simulink model "DynamicModel"  (R2022b)
settings: Solver=VariableStepAuto  StartTime=0.0  StopTime=t  FixedStep=t / k
values from neighbouring files (symbols this model uses):
  dq_0 = zeros(3, 1)    [USA_WPI.m]
  I1_n = 0.5 * (I1_n + I1_n')    [USA_WPI.m]
  I2_n = 0.5 * (I2_n + I2_n')    [USA_WPI.m]
  I3_n = 0.5 * (I3_n + I3_n')    [USA_WPI.m]
  Kp = 10 * eye(3)    [USA_WPI.m]
  L_n = [0 0.64 0.96]    [USA_WPI.m]
  Lcom_n = L_n / 2    [USA_WPI.m]
  m_n = [29.1735 40.0393 22.3124]    [USA_WPI.m]
  q_0 = randn(3, 1)    [USA_WPI.m]
settings Model: Creator=mluser  LastModifiedBy=Gary-pc
settings DataIOCC: ExternalInput=q1_s, q2_s, q3_s, dq1_s, dq2_s, dq3_s, ddq1_s, ddq2_s, ddq3_s  LoadExternalInput=on  SaveOutput=off  SignalLogging=off  DSMLogging=off  SaveTime=off  ReturnWorkspaceOutputs=off
settings ModelReferenceCC: EnableRefExpFcnMdlSchedulingChecks=on

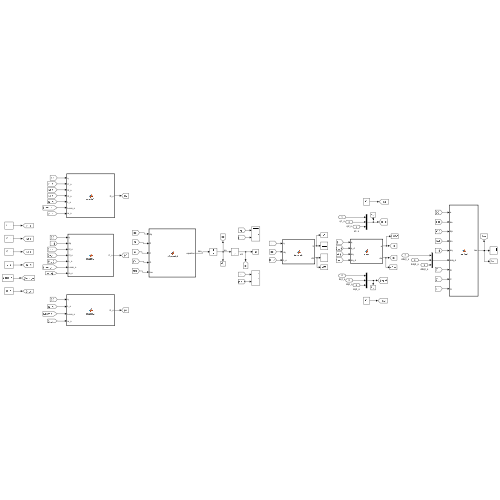
[thumbnail: Simulink's stored preview of the top-level diagram]
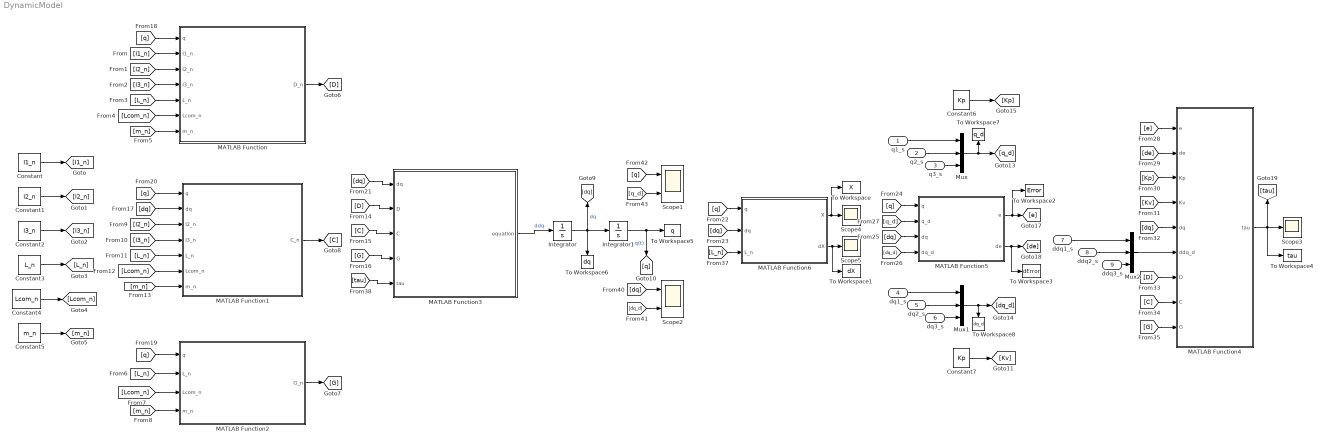
== system DynamicModel ==
  q1_s : Inport
  q2_s : Inport  Port=2
  q3_s : Inport  Port=3
  dq1_s : Inport  Port=4
  dq2_s : Inport  Port=5
  dq3_s : Inport  Port=6
  ddq1_s : Inport  Port=7
  ddq2_s : Inport  Port=8
  ddq3_s : Inport  Port=9
  Constant : Constant  Value=I1_n
  Constant1 : Constant  Value=I2_n
  Constant2 : Constant  Value=I3_n
  Constant3 : Constant  Value=L_n
  Constant4 : Constant  Value=Lcom_n
  Constant5 : Constant  Value=m_n
  Constant6 : Constant  Value=Kp
  Constant7 : Constant  Value=Kp
  Integrator : Integrator  InitialCondition=dq_0
  Integrator1 : Integrator  InitialCondition=q_0
  MATLAB Function : MATLAB Function  TreatAsAtomicUnit=on
  MATLAB Function1 : MATLAB Function  TreatAsAtomicUnit=on
  MATLAB Function2 : MATLAB Function  TreatAsAtomicUnit=on
  MATLAB Function3 : MATLAB Function  TreatAsAtomicUnit=on
  MATLAB Function4 : MATLAB Function  TreatAsAtomicUnit=on
  MATLAB Function5 : MATLAB Function  TreatAsAtomicUnit=on
  MATLAB Function6 : MATLAB Function  TreatAsAtomicUnit=on
  Mux : Mux  Inputs=3
  Mux1 : Mux  Inputs=3
  Mux2 : Mux  Inputs=3
  Scope1 : Scope  NumInputPorts=2
  Scope2 : Scope  NumInputPorts=2
  Scope3 : Scope
  Scope4 : Scope
  Scope5 : Scope
  To Workspace : ToWorkspace  VariableName=X  SaveFormat=Timeseries  SampleTime=-1
  To Workspace1 : ToWorkspace  VariableName=dX  SaveFormat=Timeseries  SampleTime=-1
  To Workspace2 : ToWorkspace  VariableName=Error  SaveFormat=Timeseries  SampleTime=-1
  To Workspace3 : ToWorkspace  VariableName=dError  SaveFormat=Timeseries  SampleTime=-1
  To Workspace4 : ToWorkspace  VariableName=tau  SaveFormat=Timeseries  SampleTime=-1
  To Workspace5 : ToWorkspace  VariableName=q  SaveFormat=Timeseries  SampleTime=-1
  To Workspace6 : ToWorkspace  VariableName=dq  SaveFormat=Timeseries  SampleTime=-1
  To Workspace7 : ToWorkspace  VariableName=q_d  SaveFormat=Timeseries  SampleTime=-1
  To Workspace8 : ToWorkspace  VariableName=dq_d  SaveFormat=Timeseries  SampleTime=-1
  wires:
  Integrator/1 -> To Workspace6/1, [dq], Integrator1/1  "dq"
  Integrator1/1 -> To Workspace5/1, [q]  "q(t)"
  Constant/1 -> [I1_n]
  Constant1/1 -> [I2_n]
  Constant2/1 -> [I3_n]
  Constant3/1 -> [L_n]
  Constant4/1 -> [Lcom_n]
  Constant5/1 -> [m_n]
  [I1_n] -> MATLAB Function/2(I1_n)
  [I2_n] -> MATLAB Function/3(I2_n)
  [I3_n] -> MATLAB Function/4(I3_n)
  [L_n] -> MATLAB Function/5(L_n)
  [Lcom_n] -> MATLAB Function/6(Lcom_n)
  [m_n] -> MATLAB Function/7(m_n)
  [I2_n] -> MATLAB Function1/3(I2_n)
  [I3_n] -> MATLAB Function1/4(I3_n)
  [L_n] -> MATLAB Function1/5(L_n)
  [Lcom_n] -> MATLAB Function1/6(Lcom_n)
  [m_n] -> MATLAB Function1/7(m_n)
  MATLAB Function3/1(equation) -> Integrator/1  "ddq"
  MATLAB Function/1(D_n) -> [D]
  MATLAB Function2/1(G_n) -> [G]
  MATLAB Function1/1(C_n) -> [C]
  [D] -> MATLAB Function3/2(D)
  [C] -> MATLAB Function3/3(C)
  [G] -> MATLAB Function3/4(G)
  [dq] -> MATLAB Function1/2(dq)
  [q] -> MATLAB Function/1(q)
  [q] -> MATLAB Function1/1(q)
  [dq] -> MATLAB Function3/1(dq)
  [q] -> MATLAB Function2/1(q)
  [L_n] -> MATLAB Function2/2(L_n)
  [Lcom_n] -> MATLAB Function2/3(Lcom_n)
  [m_n] -> MATLAB Function2/4(m_n)
  [q] -> MATLAB Function5/1(q)
  [dq] -> MATLAB Function5/3(dq)
  [dq_d] -> MATLAB Function5/4(dq_d)
  [q_d] -> MATLAB Function5/2(q_d)
  MATLAB Function5/1(e) -> To Workspace2/1, [e]
  MATLAB Function5/2(de) -> To Workspace3/1, [de]
  [e] -> MATLAB Function4/1(e)
  [de] -> MATLAB Function4/2(de)
  [Kp] -> MATLAB Function4/3(Kp)
  [Kv] -> MATLAB Function4/4(Kv)
  [dq] -> MATLAB Function4/5(dq)
  [D] -> MATLAB Function4/7(D)
  [C] -> MATLAB Function4/8(C)
  [G] -> MATLAB Function4/9(G)
  [tau] -> MATLAB Function3/5(tau)
  [dq] -> Scope2/1
  [dq_d] -> Scope2/2
  [q] -> Scope1/1
  [q_d] -> Scope1/2
  MATLAB Function4/1(tau) -> To Workspace4/1, Scope3/1, [tau]
  q1_s/1 -> Mux/1
  q2_s/1 -> Mux/2
  q3_s/1 -> Mux/3
  Mux/1 -> To Workspace7/1, [q_d]
  dq3_s/1 -> Mux1/3
  dq1_s/1 -> Mux1/1
  dq2_s/1 -> Mux1/2
  ddq2_s/1 -> Mux2/2
  ddq1_s/1 -> Mux2/1
  Mux2/1 -> MATLAB Function4/6(ddq_d)
  ddq3_s/1 -> Mux2/3
  Constant6/1 -> [Kp]
  Constant7/1 -> [Kv]
  [q] -> MATLAB Function6/1(q)
  [L_n] -> MATLAB Function6/3(L_n)
  [dq] -> MATLAB Function6/2(dq)
  MATLAB Function6/1(X) -> To Workspace/1, Scope4/1
  MATLAB Function6/2(dX) -> To Workspace1/1, Scope5/1
  Mux1/1 -> To Workspace8/1, [dq_d]

== matlab function DynamicModel/MATLAB Function1 ==
  data: C_n output; q input; dq input; I2_n input; I3_n input; L_n input; Lcom_n input; m_n input
function C_n = matrixC(q, dq, I2_n, I3_n, L_n, Lcom_n, m_n)

%% Evaluate anonymous function
C_n = functionC(I2_n(1, 1), ...
                I3_n(1, 1), ...
                I2_n(1, 2), ...
                I3_n(1, 2), ...
                I2_n(1, 3), ...
                I3_n(1, 3), ...
                I2_n(2, 2), ...
                I3_n(2, 2), ...
                I2_n(2, 3), ...
                I3_n(2, 3), ...
                I2_n(3, 3), ...
                I3_n(3, 3), ...
                L_n(2), Lcom_n(2), Lcom_n(3), dq(1), dq(2), dq(3), m_n(2), m_n(3), q(1), q(2), q(3));

== matlab function DynamicModel/MATLAB Function ==
  data: D_n output; q input; I1_n input; I2_n input; I3_n input; L_n input; Lcom_n input; m_n input
function D_n = matrixD(q, I1_n, I2_n, I3_n, L_n, Lcom_n, m_n)

%% Evaluate anonymous function
D_n = functionD(I2_n(1, 1), ...
                I3_n(1, 1), ...
                I2_n(1, 2), ...
                I3_n(1, 2), ...
                I2_n(1, 3), ...
                I3_n(1, 3), ...
                I2_n(2, 2), ...
                I3_n(2, 2), ...
                I2_n(2, 3), ...
                I3_n(2, 3), ...
                I1_n(3, 3), ...
                I2_n(3, 3), ...
                I3_n(3, 3), ...
                L_n(2), ...
                Lcom_n(2), Lcom_n(3), m_n(2), m_n(3), q(1), q(2), q(3));

== matlab function DynamicModel/MATLAB Function2 ==
  data: G_n output; q input; L_n input; Lcom_n input; m_n input
function G_n = matrixG(q, L_n, Lcom_n, m_n)

%% Evaluate anonymous function
G_n = functionG(L_n(2), Lcom_n(2), Lcom_n(3), m_n(2), m_n(3), q(2), q(3));

== matlab function DynamicModel/MATLAB Function3 ==
  data: dq input; equation output; D input; C input; G input; tau input
function equation = differential(dq, D, C, G, tau)

equation = pinv(D) * (tau - C * dq - G);

== matlab function DynamicModel/MATLAB Function4 ==
  data: e input; de input; Kp input; Kv input; dq input; ddq_d input; tau output; D input; C input; G input
function tau = control(e, de, Kp, Kv, dq, ddq_d, D, C, G)

%% Control function
tau = D * ((Kp * e) + (Kv * de) + ddq_d) + (C * dq) + G;

== matlab function DynamicModel/MATLAB Function5 ==
  data: q input; q_d input; dq input; e output; dq_d input; de output
function [e, de] = error(q, q_d, dq, dq_d)

%% Error calculation
e = q_d - q;
de = dq_d - dq;

== matlab function DynamicModel/MATLAB Function6 ==
  data: q input; dq input; X output; L_n input; dX output
function [X, dX] = forwardK(q, dq, L_n)

%% Parámetros Denavit - Hartenberg

DH = denavitHartenberg(q, L_n);

%% Cinemática Directa

% Parámetros: DH y m (marcos de referencia por analizar)
H = forwardKinematicsDH(DH, 3 + 1);

% Transforma al vector Axis - Angle
X = axisAngle(H);

%% Cinemática Diferencial

% Matriz Jacobiana Geométrica
J = jacobianMatrix(DH, q);

% Velocidad en el efector final
dX = J * dq;
